simulink model "missile_block_diagrams"  (R2023b)
settings: Solver=VariableStepAuto  StartTime=0.0  StopTime=10.0  RelTol=1e-3
values from neighbouring files (symbols this model uses):
  desiredPitch = 60    [missile_proj_variables.m]
  eta_damping = 100    [missile_proj_variables.m]
  eta_nat_freq = 250    [missile_proj_variables.m]
  K_a = 5    [missile_proj_variables.m]
  k_motor = 0.38518    [missile_proj_variables.m]
  partial_M_eta = -3    [missile_proj_variables.m]
  partial_M_q = -3    [missile_proj_variables.m]
  tau_motor = 0.6459    [missile_proj_variables.m]
settings Model: Creator=n8dsa  LastModifiedBy=n8dsa

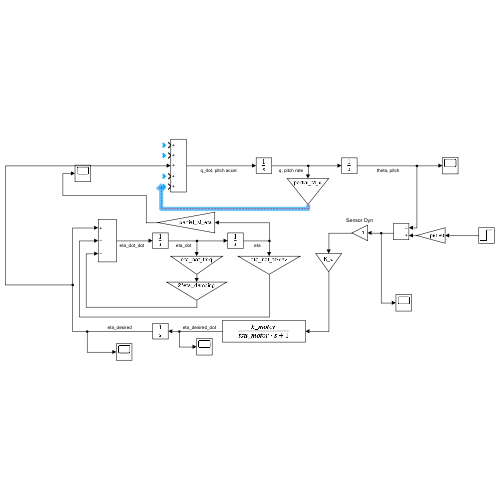
[thumbnail: Simulink's stored preview of the top-level diagram]
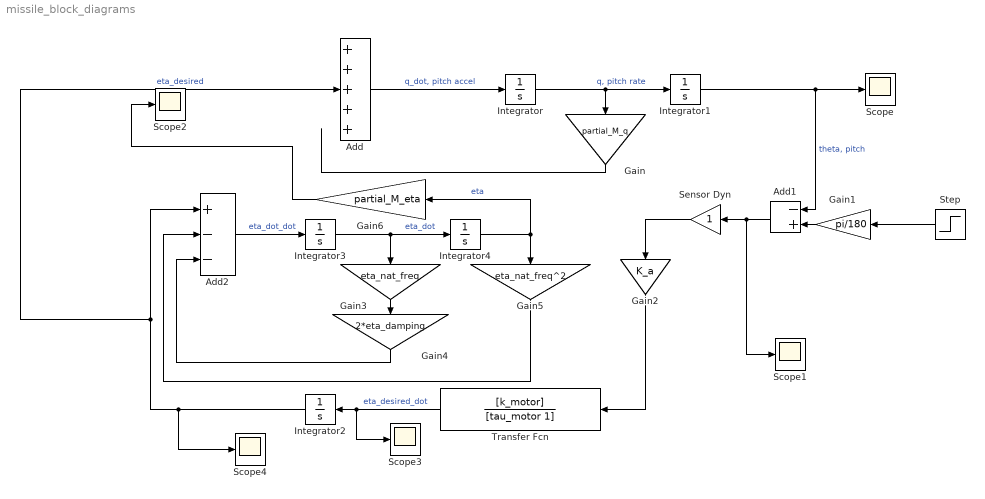
== system missile_block_diagrams ==
  Add : Sum  Inputs=+++++
  Add1 : Sum  Inputs=-+
  Add2 : Sum  Inputs=+--
  Gain : Gain  Gain=partial_M_q
  Gain1 : Gain  Gain=pi/180
  Gain2 : Gain  Gain=K_a
  Gain3 : Gain  Gain=eta_nat_freq
  Gain4 : Gain  Gain=2*eta_damping
  Gain5 : Gain  Gain=eta_nat_freq^2
  Gain6 : Gain  Gain=partial_M_eta
  Integrator{,1..4} (5 alike) : Integrator
  Scope{,1..4} (5 alike) : Scope
  Sensor Dyn : Gain
  Step : Step  Time=0.1  After=desiredPitch  SampleTime=0
  Transfer Fcn : TransferFcn  Numerator=[k_motor]  Denominator=[tau_motor 1]
  wires:
  Add/1 -> Integrator/1  "q_dot, pitch accel"
  Integrator/1 -> Gain/1, Integrator1/1  "q, pitch rate"
  Integrator1/1 -> Scope/1, Add1/1  "theta, pitch"
  Gain/1 -> ?
  Gain1/1 -> Add1/2
  Add1/1 -> Scope1/1, Sensor Dyn/1
  Sensor Dyn/1 -> Gain2/1
  Gain2/1 -> Transfer Fcn/1
  Transfer Fcn/1 -> Scope3/1, Integrator2/1  "eta_desired_dot"
  Integrator2/1 -> Scope4/1, Add/3, Add2/1  "eta_desired"
  Add2/1 -> Integrator3/1  "eta_dot_dot"
  Integrator3/1 -> Gain3/1, Integrator4/1  "eta_dot"
  Integrator4/1 -> Gain6/1, Gain5/1  "eta"
  Gain3/1 -> Gain4/1
  Gain4/1 -> Add2/3
  Gain5/1 -> Add2/2
  Gain6/1 -> Scope2/1
  Step/1 -> Gain1/1
